simulink model "electricVehicle_start"  (R2020a)
settings: Solver=ode23t  StartTime=0.0  StopTime=1000  RelTol=1e-3  AbsTol=1e-3  EnableMultiTasking=on
PreLoadFcn:
  | car_tire_data
  | load engine_data
values from neighbouring files (symbols this model uses):
  rider_mass = 80    [car_tire_data.m]
  tire_dia = 18    [car_tire_data.m]
  vehicle_mass = 237    [car_tire_data.m]
libraries: fl_lib x116, nesl_utility x16, sdl_lib x6, ee_lib x2, simulink x2, fl_ps_legacy_lib x2
(part 2 of 2)

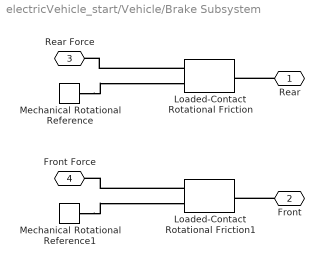
== system electricVehicle_start/Vehicle/Brake Subsystem ==
  Loaded-Contact Rotational Friction : sdl_lib/Brakes & Detents/Rotational/Loaded-Contact Rotational Friction  geometry_model=1  r_eff=280 mm  d_o=150 mm  d_i=100 mm  friction_model=1  mu_w_vector=[ 0 0.1 0.2 0.3 0.4 0.5 1 2 5 10 100 1000 ] rad/s  temperature_TLU=[280, 300, 320] K  mu_static=0.35  mu_static_vector=[.4, .38, .36]  mu_coulomb=0.3  mu_coulomb_vector=[ 0.29 0.28 0.26 0.22 0.21 0.2 0.2 0.19 0.19 0.19 0.19 0.19 ]  mu_coulomb_temp_vector=[.3, .28, .25]  mu_coulomb_matrix=[.34, .32, .3; .3, .28, .25; .25, .2, .15]  mu_interp_method=1  mu_extrap_method=1  w_tol=0.001 rad/s  force_min=1 N  mu_visc=0 N*m/(rad/s)  initial_state_locked=0  thermal_mass=50 kJ/K  T_init=300 K
      settings: SourceProductBaseCode=LD  InternalSimscapePortConfiguration="{\"Bottom\":[],\"Left\":[{\"id\":\"N\",\"label\":\"N\",\"type\":\"input\"},{\"id\":\"B\",\"label\":\"B\",\"type\":\"foundation.mechanical.rotational.rotational\"}],\"Right\":[{\"id\":\"F\",\"label\":\"F\",\"type\":\"foundation.mechanical.rotational.rotational\"}],\"Top\":[]}"
  Loaded-Contact Rotational Friction1 : sdl_lib/Brakes & Detents/Rotational/Loaded-Contact Rotational Friction  geometry_model=1  r_eff=280 mm  d_o=150 mm  d_i=100 mm  friction_model=1  mu_w_vector=[ 0 0.1 0.2 0.3 0.4 0.5 1 2 5 10 100 1000 ] rad/s  temperature_TLU=[280, 300, 320] K  mu_static=0.35  mu_static_vector=[.4, .38, .36]  mu_coulomb=0.3  mu_coulomb_vector=[ 0.29 0.28 0.26 0.22 0.21 0.2 0.2 0.19 0.19 0.19 0.19 0.19 ]  mu_coulomb_temp_vector=[.3, .28, .25]  mu_coulomb_matrix=[.34, .32, .3; .3, .28, .25; .25, .2, .15]  mu_interp_method=1  mu_extrap_method=1  w_tol=0.001 rad/s  force_min=1 N  mu_visc=0 N*m/(rad/s)  initial_state_locked=0  thermal_mass=50 kJ/K  T_init=300 K
      settings: SourceProductBaseCode=LD  InternalSimscapePortConfiguration="{\"Bottom\":[],\"Left\":[{\"id\":\"N\",\"label\":\"N\",\"type\":\"input\"},{\"id\":\"B\",\"label\":\"B\",\"type\":\"foundation.mechanical.rotational.rotational\"}],\"Right\":[{\"id\":\"F\",\"label\":\"F\",\"type\":\"foundation.mechanical.rotational.rotational\"}],\"Top\":[]}"
  Mechanical Rotational Reference : fl_lib/Mechanical/Rotational Elements/Mechanical Rotational Reference
  Mechanical Rotational Reference1 : fl_lib/Mechanical/Rotational Elements/Mechanical Rotational Reference
  Rear : PMIOPort  Side=Right
  Front : PMIOPort  Port=2  Side=Right
  Rear Force : PMIOPort  Port=3  Side=Left
  Front Force : PMIOPort  Port=4  Side=Left
  connections:
  Mechanical Rotational Reference/LConn1 -- Loaded-Contact Rotational Friction/LConn2
  Mechanical Rotational Reference1/LConn1 -- Loaded-Contact Rotational Friction1/LConn2
  Loaded-Contact Rotational Friction/LConn1 -- Rear Force/RConn1
  Loaded-Contact Rotational Friction1/LConn1 -- Front Force/RConn1
  Rear/RConn1 -- Loaded-Contact Rotational Friction/RConn1
  Front/RConn1 -- Loaded-Contact Rotational Friction1/RConn1

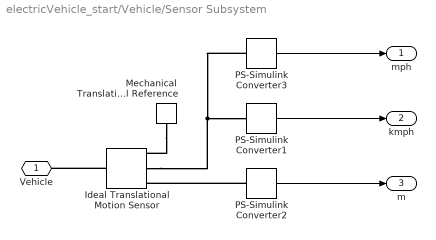
== system electricVehicle_start/Vehicle/Sensor Subsystem ==
  Ideal Translational Motion Sensor : fl_lib/Mechanical/Mechanical Sensors/Ideal Translational Motion Sensor  offset=0 m
  Mechanical Translational Reference : fl_lib/Mechanical/Translational Elements/Mechanical Translational Reference
  PS-Simulink Converter1 : nesl_utility/PS-Simulink Converter  PhysicalDomain=network_engine_domain  SubClassName=ps_output  LeftPortType=input  RightPortType=output  PseudoPeriodic=off  Frequencies=[]  Unit=km/hr  AffineConversion=off
  PS-Simulink Converter2 : nesl_utility/PS-Simulink Converter  PhysicalDomain=network_engine_domain  SubClassName=ps_output  LeftPortType=input  RightPortType=output  PseudoPeriodic=off  Frequencies=[]  Unit=1  AffineConversion=off
  PS-Simulink Converter3 : nesl_utility/PS-Simulink Converter  PhysicalDomain=network_engine_domain  SubClassName=ps_output  LeftPortType=input  RightPortType=output  PseudoPeriodic=off  Frequencies=[]  Unit=mph  AffineConversion=off
  Vehicle : PMIOPort  Side=Left
  mph : Outport  VectorParamsAs1DForOutWhenUnconnected=off
  kmph : Outport  Port=2  VectorParamsAs1DForOutWhenUnconnected=off
  m : Outport  Port=3  VectorParamsAs1DForOutWhenUnconnected=off
  wires:
  PS-Simulink Converter1/1 -> kmph/1
  PS-Simulink Converter2/1 -> m/1
  PS-Simulink Converter3/1 -> mph/1
  connections:
  Mechanical Translational Reference/LConn1 -- Ideal Translational Motion Sensor/RConn1
  PS-Simulink Converter2/LConn1 -- Ideal Translational Motion Sensor/RConn3
  Ideal Translational Motion Sensor/RConn2 -- PS-Simulink Converter3/LConn1 -- PS-Simulink Converter1/LConn1
  Ideal Translational Motion Sensor/LConn1 -- Vehicle/RConn1

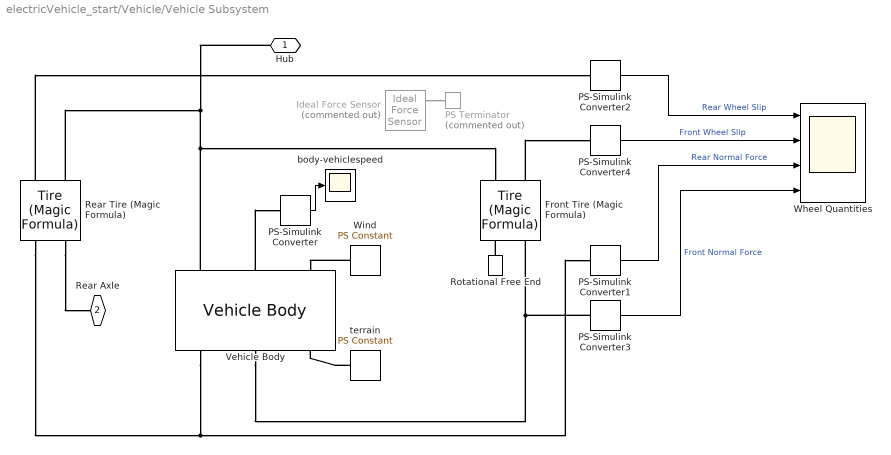
== system electricVehicle_start/Vehicle/Vehicle Subsystem ==
  Front Tire (Magic Formula) : sdl_lib/Tires & Vehicles/Tire (Magic Formula)  parameterization=2  F_z1=3e+3 N  F_x1=3.5e+3 N  kappa1=10  B_m=tire_b  C_m=tire_c  D_m=tire_d  E_m=tire_e  fz0=4e+3 N  p_Cx=1.685  p_Dx=[ 1.21 -0.037 ]  p_Ex=[ 0.344 0.095 -0.02 0 ]  p_Kx=[ 21.51 -0.163 0.245 ]  p_Hx=[ -0.002 0.002 ]  p_Vx=[ 0 0 ]  v_tr_thr=0.1 m/s  r_e=tire_dia/2 in  model_compliance=0  stiffness=1e+6 N/m  damping=1000 N/(m/s)  model_inertia=1  inertia=tire_inertia kg*m^2  initial_velocity=0 rad/s  model_resistance=1  resistance_model=1  coeff=roll_resist  p_tire=250e3 Pa  alpha=-0.003  beta=0.97  coeff_a=84e-4  coeff_b=6.2e-4 s/m  coeff_c=1.6e-4 s^2/m^2  v_thr=1e-3 m/s
  Ideal Force Sensor : fl_lib/Mechanical/Mechanical Sensors/Ideal Force Sensor  Commented=on
  PS Terminator : fl_lib/Physical Signals/Sinks/PS Terminator  Commented=on
  PS-Simulink Converter : nesl_utility/PS-Simulink Converter  PhysicalDomain=network_engine_domain  SubClassName=ps_output  LeftPortType=input  RightPortType=output  PseudoPeriodic=off  Frequencies=[]  Unit=km/hr  AffineConversion=off
  PS-Simulink Converter{1..4} (4 alike) : nesl_utility/PS-Simulink Converter  PhysicalDomain=network_engine_domain  SubClassName=ps_output  LeftPortType=input  RightPortType=output  PseudoPeriodic=off  Frequencies=[]  Unit=N  AffineConversion=off
  Rear Tire (Magic Formula) : sdl_lib/Tires & Vehicles/Tire (Magic Formula)  parameterization=2  F_z1=3e+3 N  F_x1=3.5e+3 N  kappa1=10  B_m=tire_b  C_m=tire_c  D_m=tire_d  E_m=tire_e  fz0=4e+3 N  p_Cx=1.685  p_Dx=[ 1.21 -0.037 ]  p_Ex=[ 0.344 0.095 -0.02 0 ]  p_Kx=[ 21.51 -0.163 0.245 ]  p_Hx=[ -0.002 0.002 ]  p_Vx=[ 0 0 ]  v_tr_thr=0.1 m/s  r_e=tire_dia/2 in  model_compliance=0  stiffness=1e+6 N/m  damping=1000 N/(m/s)  model_inertia=1  inertia=tire_inertia kg*m^2  initial_velocity=0 rad/s  model_resistance=1  resistance_model=1  coeff=roll_resist  p_tire=250e3 Pa  alpha=-0.003  beta=0.97  coeff_a=84e-4  coeff_b=6.2e-4 s/m  coeff_c=1.6e-4 s^2/m^2  v_thr=1e-3 m/s
  Rotational Free End : fl_lib/Mechanical/Rotational Elements/Rotational Free End  w_specify=off  w_priority=None  w=0 rad/s  w_nominal_specify=off  w_nominal_unit=rad/s  w_nominal_value=1
      settings: SourceProductBaseCode=SS
  Vehicle Body : sdl_lib/Tires & Vehicles/Vehicle Body  mass=rider_mass + vehicle_mass kg  n_w=1  x_f=front_axle mm  x_r=rear_axle mm  y_c=CG_height mm  mass_var=simscape.enum.onoff.off  model_pitch=simscape.enum.onoff.on  inertia=4000 kg*m^2  suspension_model=sdl.enum.linearTLU.linear  k_f=1e4 N/m  b_f=1e4 N/(m/s)  k_r=1e4 N/m  b_r=1e4 N/(m/s)  k_f_TLU=[-2000, -1000, 0, 1000, 2000] N  x_f_TLU=[-.4, -.2, 0, .2, .4] m  b_f_TLU=[-200, -100, 0, 100, 200] N  v_f_TLU=[-4, -2, 0, 2, 4] m/s  k_r_TLU=[-2000, -1000, 0, 1000, 2000] N  x_r_TLU=[-.4, -.2, 0, .2, .4] m  b_r_TLU=[-200, -100, 0, 100, 200] N  v_r_TLU=[-4, -2, 0, 2, 4] m/s  interp_method=simscape.enum.interpolation.linear  extrap_method=simscape.enum.extrapolation.linear  model_hardstop=simscape.enum.onoff.off  upper_bound_f=.25 m  lower_bound_f=-.25 m  stop_k_f=1e6 N/m  stop_b_f=150 N/(m/s)  upper_bound_r=.25 m  lower_bound_r=-.25 m  stop_k_r=1e6 N/m  stop_b_r=150 N/(m/s)  initial_pitch=0 rad  initial_pitch_rate=0 rad/s  g=9.81 m/s^2  liftoff_warning=simscape.enum.onoff.off  area=front_area m^2  Cd=drag_coeff  rho=1.18 kg/m^3  v_specify=on  v_priority=High  v=0 m/s  v_nominal_specify=off  v_nominal_unit=m/s  v_nominal_value=1
  Wheel Quantities : Scope  NumInputPorts=4
  Wind : fl_lib/Physical Signals/Sources/PS Constant  constant=10 km/hr
  body-vehiclespeed : Scope
  terrain : fl_lib/Physical Signals/Sources/PS Constant  constant=0*(pi/180) rad
  Hub : PMIOPort  Side=Right
  Rear Axle : PMIOPort  Port=2  Side=Left
  wires:
  PS-Simulink Converter/1 -> body-vehiclespeed/1
  PS-Simulink Converter2/1 -> Wheel Quantities/1  "Rear Wheel Slip"
  PS-Simulink Converter4/1 -> Wheel Quantities/2  "Front Wheel Slip"
  PS-Simulink Converter1/1 -> Wheel Quantities/3  "Rear Normal Force"
  PS-Simulink Converter3/1 -> Wheel Quantities/4  "Front Normal Force"
  connections:
  Vehicle Body/RConn1 -- Rear Tire (Magic Formula)/LConn1 -- PS-Simulink Converter1/LConn1
  Front Tire (Magic Formula)/LConn1 -- Vehicle Body/RConn2 -- PS-Simulink Converter3/LConn1
  Vehicle Body/LConn2 -- PS-Simulink Converter/LConn1
  Rear Tire (Magic Formula)/RConn2 -- Vehicle Body/LConn1 -- Front Tire (Magic Formula)/RConn2 -- Hub/RConn1
  Rear Tire (Magic Formula)/LConn2 -- Rear Axle/RConn1
  Rotational Free End/LConn1 -- Front Tire (Magic Formula)/LConn2
  Front Tire (Magic Formula)/RConn1 -- PS-Simulink Converter4/LConn1
  Rear Tire (Magic Formula)/RConn1 -- PS-Simulink Converter2/LConn1
  Ideal Force Sensor/RConn2 -- PS Terminator/LConn1
  Wind/RConn1 -- Vehicle Body/LConn3
  terrain/RConn1 -- Vehicle Body/RConn3
